simulink model "TSR_Scenario_003_cs"  (R2014b)
settings: Solver=ode5  SolverMode=SingleTasking  StartTime=0.0  StopTime=inf  FixedStep=1/100  RelTol=1e-3
PreLoadFcn:
  | mbxruntime.callbacks.PreLoadFcn(bdroot);
  | check_NUTS_defined;
  | 
  | assignin('base',['model_closed_' bdroot],false);
  | 
  | addpath('../includes_TSR/includes_TSR');
  | 
  | switch version('-release')
  | case {'2010a', '2010b', '2011a'}
  | addpath('../includes_TSR/ML2010b');
  | otherwise
  | addpath('../includes_TSR/ML2011b');
  | end
PostLoadFcn:
  | mbxruntime.callbacks.PostLoadFcn(bdroot);
InitFcn:
  | mbxruntime.callbacks.InitFcn(bdroot);
StartFcn:
  | mbxruntime.callbacks.StartFcn(bdroot);
StopFcn:
  | mbxruntime.callbacks.StopFcn(bdroot);
model workspace: external: MAT-File .\TSR_Scenario_003_cs_hws.mat (data not in the file)
undefined symbols (not defined in the file or in its folder): InitImageOutputDir, mbxruntime, OrientationPitch, OrientationRoll, PositionX, PositionY, PositionZ, tabledata, warningInitialVelocity, x0
undefined symbols (not defined in the file): SteeringColumn, SteeringWheel, TSR_Scenario_003_cs_031c08980fc50484, TSR_Scenario_003_cs_034f292ed02288d5, TSR_Scenario_003_cs_0459b3dfbc82c9a8, TSR_Scenario_003_cs_097620f815f21f1d, TSR_Scenario_003_cs_097d7573cc694bf5, TSR_Scenario_003_cs_0996a1a3dd5e2a3a, TSR_Scenario_003_cs_0f1849cdb4701326, TSR_Scenario_003_cs_10f4098912b3b5db, TSR_Scenario_003_cs_117f01ea831ec368, TSR_Scenario_003_cs_12cf78b79d36da1c, TSR_Scenario_003_cs_144fbb977118bf37, TSR_Scenario_003_cs_1523d5367c5052d0, TSR_Scenario_003_cs_1540f37e1ce5220e, TSR_Scenario_003_cs_15da4682074a9114, TSR_Scenario_003_cs_186e86d78e8adde8, TSR_Scenario_003_cs_198fefcb5c5d4c4a, TSR_Scenario_003_cs_1d24564a28ca8c57, TSR_Scenario_003_cs_1ea9b65b93b2d93e, TSR_Scenario_003_cs_1f4a4c0163bc654f, TSR_Scenario_003_cs_221c7f4f757b6f59, TSR_Scenario_003_cs_22229c9f69845439, TSR_Scenario_003_cs_230bf92302b3240a, TSR_Scenario_003_cs_23763ac742803108, TSR_Scenario_003_cs_237ee3c37f4d72b6, TSR_Scenario_003_cs_2956d712ba1268bc, TSR_Scenario_003_cs_2c8e6bdc42e74688, TSR_Scenario_003_cs_3037724928f99df0, TSR_Scenario_003_cs_31b44ca47ec5ff02, TSR_Scenario_003_cs_324745b613f45b9c, TSR_Scenario_003_cs_32b36e3fd4699b17, TSR_Scenario_003_cs_35d6077a5f3bdf8f, TSR_Scenario_003_cs_364710b5c901cafc, TSR_Scenario_003_cs_3727ee2f4430f2bb, TSR_Scenario_003_cs_382e41ab6806a13f, TSR_Scenario_003_cs_38ccddae174883be, TSR_Scenario_003_cs_3a0767dbf486e31b, TSR_Scenario_003_cs_3b460d19c10c747b, TSR_Scenario_003_cs_426c63b9f9c7abdf, TSR_Scenario_003_cs_42f1edf1b324bf4e, TSR_Scenario_003_cs_43b33e682c00a164, TSR_Scenario_003_cs_440a2f0d77aab01b, TSR_Scenario_003_cs_466378c5e179d625, TSR_Scenario_003_cs_4b8aa743d5bd8c1e, TSR_Scenario_003_cs_4bb095d5f4984042, TSR_Scenario_003_cs_4cec1a92176fe53d, TSR_Scenario_003_cs_4d6b6c843c52af2c, TSR_Scenario_003_cs_514fc139d324fd0d, TSR_Scenario_003_cs_51f4eff9e91179f9, TSR_Scenario_003_cs_56a9ea09cd860a89, TSR_Scenario_003_cs_5749c15298076949, TSR_Scenario_003_cs_576a8029b2a2792f, TSR_Scenario_003_cs_58b2f104991e8ca9, TSR_Scenario_003_cs_59a8a0af3bc025d5, TSR_Scenario_003_cs_5baf0e640050f43b, TSR_Scenario_003_cs_626299c795c4a86e, TSR_Scenario_003_cs_6499aa317499632d, TSR_Scenario_003_cs_676e881463a7df3e, TSR_Scenario_003_cs_68379cf1a8816ef6 ... (+115)
libraries: PreScanSimulinkLibrary x53, simulink_extras x37, simulink x29
(part 3 of 21)

== system TSR_Scenario_003_cs/Audi_A8_1_Indicator_front_right ==
  Audi_A8_1_Indicator_front_right : Inport  Tag=inport/IndicatorFR  OutDataTypeStr=Bus: PRESCAN_VISULIGHTACTUATOR_DATA  SampleTime=1/100  BusOutputAsStruct=on
  Actuator : S-Function  FunctionName=sfun_VisuLightActuator  Parameters=mbxruntime.parameters.convert(UniqueID), mbxruntime.parameters.convert(LightName), mbxruntime.parameters.convert(PivotName), mbxruntime.parameters.convert(TextureResources), mbxruntime.parameters.convert(ColorsObjectName), mbxruntime.parameters.convert(MeshOnColor), mbxruntime.parameters.convert(MeshOffColor),tabledata, TimeStep  EnableBusSupport=off  mask(PreScan Sink Block: VisuActiveLight){UniqueID=210, LightName=Audi_A8_1.LightActuator_8_IndicatorFR_ActiveLight, PivotName=Audi_A8_1.IndicatorFR_pivot, TextureResources={ '1' 'LightMap\HeadLight LB and HB.png' '2' 'LightMap\HeadLight LB.png' '3' 'LightMap\GeneralLight.png' '4' 'LightMap\BrakeLight.png'}, ColorsObjectName=Audi_A8_1.IndicatorFR, MeshOnColor=[255  165    0    0  255  165    0    0  102  102  102  255  510  420  178  255], MeshOffColor=[255  165    0    0  255  165    0    0  102  102  102  255    0    0    0  255], TimeStep=1/100}
      mask prompts: UniqueID "Parent Unique Identifier"; LightName "Light"; PivotName "Pivot"; TextureResources "Texture Resources"; ColorsObjectName "Light Fixture Color Object"; MeshOnColor "Light Fixture On Color"; MeshOffColor "Light Fixture Off Color"; TimeStep "Simulink time step"
      mask help:
      | The VisuActiveLight block provides a way for detailed animation of Light Sources, such as the indicator, brake, fog and main lights of a vehicle, or a light post.
      |
      | For more information, please click Help.
      mask init:
      | [tabledata] = mbxruntime.parameters.table(UniqueID,LightName,PivotName,TextureResources,ColorsObjectName,MeshOnColor,MeshOffColor);
      mask Help: eval('openHelp(209)')
      mask Display: image(imread('HeadLight.png'))
  wires:
  Audi_A8_1_Indicator_front_right/1 -> Actuator/1

== system TSR_Scenario_003_cs/Audi_A8_1_Indicator_rear_left ==
  Audi_A8_1_Indicator_rear_left : Inport  Tag=inport/IndicatorRL  OutDataTypeStr=Bus: PRESCAN_VISULIGHTACTUATOR_DATA  SampleTime=1/100  BusOutputAsStruct=on
  Actuator : S-Function  FunctionName=sfun_VisuLightActuator  Parameters=mbxruntime.parameters.convert(UniqueID), mbxruntime.parameters.convert(LightName), mbxruntime.parameters.convert(PivotName), mbxruntime.parameters.convert(TextureResources), mbxruntime.parameters.convert(ColorsObjectName), mbxruntime.parameters.convert(MeshOnColor), mbxruntime.parameters.convert(MeshOffColor),tabledata, TimeStep  EnableBusSupport=off  mask(PreScan Sink Block: VisuActiveLight){UniqueID=210, LightName=Audi_A8_1.LightActuator_7_IndicatorRL_ActiveLight, PivotName=Audi_A8_1.IndicatorRL_pivot, TextureResources={ '1' 'LightMap\HeadLight LB and HB.png' '2' 'LightMap\HeadLight LB.png' '3' 'LightMap\GeneralLight.png' '4' 'LightMap\BrakeLight.png'}, ColorsObjectName=Audi_A8_1.IndicatorRL, MeshOnColor=[255  165    0    0  255  165    0    0  102  102  102  255  510  420  178  255], MeshOffColor=[255  165    0    0  255  165    0    0  102  102  102  255    0    0    0  255], TimeStep=1/100}
      mask prompts: UniqueID "Parent Unique Identifier"; LightName "Light"; PivotName "Pivot"; TextureResources "Texture Resources"; ColorsObjectName "Light Fixture Color Object"; MeshOnColor "Light Fixture On Color"; MeshOffColor "Light Fixture Off Color"; TimeStep "Simulink time step"
      mask help:
      | The VisuActiveLight block provides a way for detailed animation of Light Sources, such as the indicator, brake, fog and main lights of a vehicle, or a light post.
      |
      | For more information, please click Help.
      mask init:
      | [tabledata] = mbxruntime.parameters.table(UniqueID,LightName,PivotName,TextureResources,ColorsObjectName,MeshOnColor,MeshOffColor);
      mask Help: eval('openHelp(209)')
      mask Display: image(imread('HeadLight.png'))
  wires:
  Audi_A8_1_Indicator_rear_left/1 -> Actuator/1

== system TSR_Scenario_003_cs/Audi_A8_1_Indicator_rear_right ==
  Audi_A8_1_Indicator_rear_right : Inport  Tag=inport/IndicatorRR  OutDataTypeStr=Bus: PRESCAN_VISULIGHTACTUATOR_DATA  SampleTime=1/100  BusOutputAsStruct=on
  Actuator : S-Function  FunctionName=sfun_VisuLightActuator  Parameters=mbxruntime.parameters.convert(UniqueID), mbxruntime.parameters.convert(LightName), mbxruntime.parameters.convert(PivotName), mbxruntime.parameters.convert(TextureResources), mbxruntime.parameters.convert(ColorsObjectName), mbxruntime.parameters.convert(MeshOnColor), mbxruntime.parameters.convert(MeshOffColor),tabledata, TimeStep  EnableBusSupport=off  mask(PreScan Sink Block: VisuActiveLight){UniqueID=210, LightName=Audi_A8_1.LightActuator_9_IndicatorRR_ActiveLight, PivotName=Audi_A8_1.IndicatorRR_pivot, TextureResources={ '1' 'LightMap\HeadLight LB and HB.png' '2' 'LightMap\HeadLight LB.png' '3' 'LightMap\GeneralLight.png' '4' 'LightMap\BrakeLight.png'}, ColorsObjectName=Audi_A8_1.IndicatorRR, MeshOnColor=[255  165    0    0  255  165    0    0  102  102  102  255  510  420  178  255], MeshOffColor=[255  165    0    0  255  165    0    0  102  102  102  255    0    0    0  255], TimeStep=1/100}
      mask prompts: UniqueID "Parent Unique Identifier"; LightName "Light"; PivotName "Pivot"; TextureResources "Texture Resources"; ColorsObjectName "Light Fixture Color Object"; MeshOnColor "Light Fixture On Color"; MeshOffColor "Light Fixture Off Color"; TimeStep "Simulink time step"
      mask help:
      | The VisuActiveLight block provides a way for detailed animation of Light Sources, such as the indicator, brake, fog and main lights of a vehicle, or a light post.
      |
      | For more information, please click Help.
      mask init:
      | [tabledata] = mbxruntime.parameters.table(UniqueID,LightName,PivotName,TextureResources,ColorsObjectName,MeshOnColor,MeshOffColor);
      mask Help: eval('openHelp(209)')
      mask Display: image(imread('HeadLight.png'))
  wires:
  Audi_A8_1_Indicator_rear_right/1 -> Actuator/1

== system TSR_Scenario_003_cs/BMW_X5_1 ==
  SELF_BMW_X5_1 : Inport  Tag=inport/SelfPort  OutDataTypeStr=Bus: PRESCAN_SELFSENSORDATA  PortDimensions=1  SampleTime=1/100  BusOutputAsStruct=on
  Dynamics_Empty : Subsystem  Tag=Dynamics_Empty
      mask Help: eval('openHelp(202)')
      mask Display: port_label('output', 1, 'State');text(0,0,' Empty\n')
  SELF_Demux : Subsystem  Tag=demux/SelfPort  mask(PreScan Demux Block:){}
      mask help:
      | The SELF port shows (state) information of the actor itself. The outputs are position in the experiment's axis system and the GPS coordinates, and the object's absolute velocity and compass heading.
      |
      | For more information, please click Help.
      settings: DeleteFcn=PreScanBlockDeleteFcn;
      mask Help: eval('openHelp(462)')
      mask Display:
      | port_label('output',1,'x [m]')
      | port_label('output',2,'y [m]')
      | port_label('output',3,'z [m]','texmode','on')
      | port_label('output',4,'Rotx [deg]','texmode','on')
      | port_label('output',5,'Roty [deg]','texmode','on')
      | port_label('output',6,'Rotz [deg]','texmode','on')
      | port_label('output',7,'GPS lat [deg]','texmode','on')
      | port_label('output',8,'GPS long [deg]','texmode','on')
      | port_label('output',9,'GPS alt [m]','texmode','on')
      | port_label('output',10,'Velocity [m/s]')
      | port_label('output',11,'Heading [deg]')
      | port_label('output',12,'Yaw rate [deg/s]')
  STATE_BMW_X5_1_rc : RateTransition  Tag=mux_rc/StatePort  OutPortSampleTimeOpt=Inherit
  Terminator_{1..12} (12 alike) : Terminator
  STATE_BMW_X5_1_bus : Outport  Tag=outport/StatePort  OutDataTypeStr=Bus: PRESCAN_STATEACTUATORDATA  PortDimensions=1  SampleTime=1/100
  wires:
  STATE_BMW_X5_1_rc/1 -> STATE_BMW_X5_1_bus/1
  Dynamics_Empty/1(State) -> STATE_BMW_X5_1_rc/1
  SELF_BMW_X5_1/1 -> SELF_Demux/1(SELF)
  SELF_Demux/1(x [m]) -> Terminator_1/1
  SELF_Demux/2(y [m]) -> Terminator_2/1
  SELF_Demux/3(z [m]) -> Terminator_3/1
  SELF_Demux/4(rotx [deg]) -> Terminator_4/1
  SELF_Demux/5(roty [deg]) -> Terminator_5/1
  SELF_Demux/6(rotz [deg]) -> Terminator_6/1
  SELF_Demux/7(GPS lat [deg]) -> Terminator_7/1
  SELF_Demux/8(GPS long [deg]) -> Terminator_8/1
  SELF_Demux/9(GPS alt [m]) -> Terminator_9/1
  SELF_Demux/10(velocity [m/s]) -> Terminator_10/1
  SELF_Demux/11(heading [deg]) -> Terminator_11/1
  SELF_Demux/12(yaw rate [deg/s]) -> Terminator_12/1

== system TSR_Scenario_003_cs/BMW_X5_2 ==
  SELF_BMW_X5_2 : Inport  Tag=inport/SelfPort  OutDataTypeStr=Bus: PRESCAN_SELFSENSORDATA  PortDimensions=1  SampleTime=1/100  BusOutputAsStruct=on
  Dynamics_Empty : Subsystem  Tag=Dynamics_Empty
      mask Help: eval('openHelp(202)')
      mask Display: port_label('output', 1, 'State');text(0,0,' Empty\n')
  SELF_Demux : Subsystem  Tag=demux/SelfPort  mask(PreScan Demux Block:){}
      mask help:
      | The SELF port shows (state) information of the actor itself. The outputs are position in the experiment's axis system and the GPS coordinates, and the object's absolute velocity and compass heading.
      |
      | For more information, please click Help.
      settings: DeleteFcn=PreScanBlockDeleteFcn;
      mask Help: eval('openHelp(462)')
      mask Display:
      | port_label('output',1,'x [m]')
      | port_label('output',2,'y [m]')
      | port_label('output',3,'z [m]','texmode','on')
      | port_label('output',4,'Rotx [deg]','texmode','on')
      | port_label('output',5,'Roty [deg]','texmode','on')
      | port_label('output',6,'Rotz [deg]','texmode','on')
      | port_label('output',7,'GPS lat [deg]','texmode','on')
      | port_label('output',8,'GPS long [deg]','texmode','on')
      | port_label('output',9,'GPS alt [m]','texmode','on')
      | port_label('output',10,'Velocity [m/s]')
      | port_label('output',11,'Heading [deg]')
      | port_label('output',12,'Yaw rate [deg/s]')
  STATE_BMW_X5_2_rc : RateTransition  Tag=mux_rc/StatePort  OutPortSampleTimeOpt=Inherit
  Terminator_{1..12} (12 alike) : Terminator
  STATE_BMW_X5_2_bus : Outport  Tag=outport/StatePort  OutDataTypeStr=Bus: PRESCAN_STATEACTUATORDATA  PortDimensions=1  SampleTime=1/100
  wires:
  STATE_BMW_X5_2_rc/1 -> STATE_BMW_X5_2_bus/1
  Dynamics_Empty/1(State) -> STATE_BMW_X5_2_rc/1
  SELF_BMW_X5_2/1 -> SELF_Demux/1(SELF)
  SELF_Demux/1(x [m]) -> Terminator_1/1
  SELF_Demux/2(y [m]) -> Terminator_2/1
  SELF_Demux/3(z [m]) -> Terminator_3/1
  SELF_Demux/4(rotx [deg]) -> Terminator_4/1
  SELF_Demux/5(roty [deg]) -> Terminator_5/1
  SELF_Demux/6(rotz [deg]) -> Terminator_6/1
  SELF_Demux/7(GPS lat [deg]) -> Terminator_7/1
  SELF_Demux/8(GPS long [deg]) -> Terminator_8/1
  SELF_Demux/9(GPS alt [m]) -> Terminator_9/1
  SELF_Demux/10(velocity [m/s]) -> Terminator_10/1
  SELF_Demux/11(heading [deg]) -> Terminator_11/1
  SELF_Demux/12(yaw rate [deg/s]) -> Terminator_12/1

== system TSR_Scenario_003_cs/BMW_X5_3 ==
  SELF_BMW_X5_3 : Inport  Tag=inport/SelfPort  OutDataTypeStr=Bus: PRESCAN_SELFSENSORDATA  PortDimensions=1  SampleTime=1/100  BusOutputAsStruct=on
  Dynamics_Empty : Subsystem  Tag=Dynamics_Empty
      mask Help: eval('openHelp(202)')
      mask Display: port_label('output', 1, 'State');text(0,0,' Empty\n')
  SELF_Demux : Subsystem  Tag=demux/SelfPort  mask(PreScan Demux Block:){}
      mask help:
      | The SELF port shows (state) information of the actor itself. The outputs are position in the experiment's axis system and the GPS coordinates, and the object's absolute velocity and compass heading.
      |
      | For more information, please click Help.
      settings: DeleteFcn=PreScanBlockDeleteFcn;
      mask Help: eval('openHelp(462)')
      mask Display:
      | port_label('output',1,'x [m]')
      | port_label('output',2,'y [m]')
      | port_label('output',3,'z [m]','texmode','on')
      | port_label('output',4,'Rotx [deg]','texmode','on')
      | port_label('output',5,'Roty [deg]','texmode','on')
      | port_label('output',6,'Rotz [deg]','texmode','on')
      | port_label('output',7,'GPS lat [deg]','texmode','on')
      | port_label('output',8,'GPS long [deg]','texmode','on')
      | port_label('output',9,'GPS alt [m]','texmode','on')
      | port_label('output',10,'Velocity [m/s]')
      | port_label('output',11,'Heading [deg]')
      | port_label('output',12,'Yaw rate [deg/s]')
  STATE_BMW_X5_3_rc : RateTransition  Tag=mux_rc/StatePort  OutPortSampleTimeOpt=Inherit
  Terminator_{1..12} (12 alike) : Terminator
  STATE_BMW_X5_3_bus : Outport  Tag=outport/StatePort  OutDataTypeStr=Bus: PRESCAN_STATEACTUATORDATA  PortDimensions=1  SampleTime=1/100
  wires:
  STATE_BMW_X5_3_rc/1 -> STATE_BMW_X5_3_bus/1
  Dynamics_Empty/1(State) -> STATE_BMW_X5_3_rc/1
  SELF_BMW_X5_3/1 -> SELF_Demux/1(SELF)
  SELF_Demux/1(x [m]) -> Terminator_1/1
  SELF_Demux/2(y [m]) -> Terminator_2/1
  SELF_Demux/3(z [m]) -> Terminator_3/1
  SELF_Demux/4(rotx [deg]) -> Terminator_4/1
  SELF_Demux/5(roty [deg]) -> Terminator_5/1
  SELF_Demux/6(rotz [deg]) -> Terminator_6/1
  SELF_Demux/7(GPS lat [deg]) -> Terminator_7/1
  SELF_Demux/8(GPS long [deg]) -> Terminator_8/1
  SELF_Demux/9(GPS alt [m]) -> Terminator_9/1
  SELF_Demux/10(velocity [m/s]) -> Terminator_10/1
  SELF_Demux/11(heading [deg]) -> Terminator_11/1
  SELF_Demux/12(yaw rate [deg/s]) -> Terminator_12/1

== system TSR_Scenario_003_cs/BMW_Z3_1 ==
  SELF_BMW_Z3_1 : Inport  Tag=inport/SelfPort  OutDataTypeStr=Bus: PRESCAN_SELFSENSORDATA  PortDimensions=1  SampleTime=1/100  BusOutputAsStruct=on
  Dynamics_Empty : Subsystem  Tag=Dynamics_Empty
      mask Help: eval('openHelp(202)')
      mask Display: port_label('output', 1, 'State');text(0,0,' Empty\n')
  SELF_Demux : Subsystem  Tag=demux/SelfPort  mask(PreScan Demux Block:){}
      mask help:
      | The SELF port shows (state) information of the actor itself. The outputs are position in the experiment's axis system and the GPS coordinates, and the object's absolute velocity and compass heading.
      |
      | For more information, please click Help.
      settings: DeleteFcn=PreScanBlockDeleteFcn;
      mask Help: eval('openHelp(462)')
      mask Display:
      | port_label('output',1,'x [m]')
      | port_label('output',2,'y [m]')
      | port_label('output',3,'z [m]','texmode','on')
      | port_label('output',4,'Rotx [deg]','texmode','on')
      | port_label('output',5,'Roty [deg]','texmode','on')
      | port_label('output',6,'Rotz [deg]','texmode','on')
      | port_label('output',7,'GPS lat [deg]','texmode','on')
      | port_label('output',8,'GPS long [deg]','texmode','on')
      | port_label('output',9,'GPS alt [m]','texmode','on')
      | port_label('output',10,'Velocity [m/s]')
      | port_label('output',11,'Heading [deg]')
      | port_label('output',12,'Yaw rate [deg/s]')
  STATE_BMW_Z3_1_rc : RateTransition  Tag=mux_rc/StatePort  OutPortSampleTimeOpt=Inherit
  Terminator_{1..12} (12 alike) : Terminator
  STATE_BMW_Z3_1_bus : Outport  Tag=outport/StatePort  OutDataTypeStr=Bus: PRESCAN_STATEACTUATORDATA  PortDimensions=1  SampleTime=1/100
  wires:
  STATE_BMW_Z3_1_rc/1 -> STATE_BMW_Z3_1_bus/1
  Dynamics_Empty/1(State) -> STATE_BMW_Z3_1_rc/1
  SELF_BMW_Z3_1/1 -> SELF_Demux/1(SELF)
  SELF_Demux/1(x [m]) -> Terminator_1/1
  SELF_Demux/2(y [m]) -> Terminator_2/1
  SELF_Demux/3(z [m]) -> Terminator_3/1
  SELF_Demux/4(rotx [deg]) -> Terminator_4/1
  SELF_Demux/5(roty [deg]) -> Terminator_5/1
  SELF_Demux/6(rotz [deg]) -> Terminator_6/1
  SELF_Demux/7(GPS lat [deg]) -> Terminator_7/1
  SELF_Demux/8(GPS long [deg]) -> Terminator_8/1
  SELF_Demux/9(GPS alt [m]) -> Terminator_9/1
  SELF_Demux/10(velocity [m/s]) -> Terminator_10/1
  SELF_Demux/11(heading [deg]) -> Terminator_11/1
  SELF_Demux/12(yaw rate [deg/s]) -> Terminator_12/1

== system TSR_Scenario_003_cs/CameraSensor_1 ==
  Sensor : S-Function  FunctionName=sfun_Camera  Parameters=sensorID, dataWidth, dataHeight, channelsPerImage, numberOfImages, timestep  EnableBusSupport=off  mask(PreScan Source Block: Camera Sensor){sensorID=239, dataWidth=600, dataHeight=2400, channelsPerImage=3, numberOfImages=1, timestep=1/50}
      mask prompts: sensorID "Sensor ID"; dataWidth "Data width"; dataHeight "Data Height"; channelsPerImage "Channels per image"; numberOfImages "Number of images"; timestep "MATLAB timestep:"
      mask help: The Camera Sensor provides a color or monochrome image.
      mask Help: eval('openHelp(457)')
      mask Display: image(imread('CameraSensor.png'))
  CameraSensor_1 : Outport  Tag=outport/Camera/CameraSensor  OutDataTypeStr=uint8  SampleTime=1/50
  wires:
  Sensor/1 -> CameraSensor_1/1

== system TSR_Scenario_003_cs/Citroen_C3_1 ==
  SELF_Citroen_C3_1 : Inport  Tag=inport/SelfPort  OutDataTypeStr=Bus: PRESCAN_SELFSENSORDATA  PortDimensions=1  SampleTime=1/100  BusOutputAsStruct=on
  Dynamics_Empty : Subsystem  Tag=Dynamics_Empty
      mask Help: eval('openHelp(202)')
      mask Display: port_label('output', 1, 'State');text(0,0,' Empty\n')
  SELF_Demux : Subsystem  Tag=demux/SelfPort  mask(PreScan Demux Block:){}
      mask help:
      | The SELF port shows (state) information of the actor itself. The outputs are position in the experiment's axis system and the GPS coordinates, and the object's absolute velocity and compass heading.
      |
      | For more information, please click Help.
      settings: DeleteFcn=PreScanBlockDeleteFcn;
      mask Help: eval('openHelp(462)')
      mask Display:
      | port_label('output',1,'x [m]')
      | port_label('output',2,'y [m]')
      | port_label('output',3,'z [m]','texmode','on')
      | port_label('output',4,'Rotx [deg]','texmode','on')
      | port_label('output',5,'Roty [deg]','texmode','on')
      | port_label('output',6,'Rotz [deg]','texmode','on')
      | port_label('output',7,'GPS lat [deg]','texmode','on')
      | port_label('output',8,'GPS long [deg]','texmode','on')
      | port_label('output',9,'GPS alt [m]','texmode','on')
      | port_label('output',10,'Velocity [m/s]')
      | port_label('output',11,'Heading [deg]')
      | port_label('output',12,'Yaw rate [deg/s]')
  STATE_Citroen_C3_1_rc : RateTransition  Tag=mux_rc/StatePort  OutPortSampleTimeOpt=Inherit
  Terminator_{1..12} (12 alike) : Terminator
  STATE_Citroen_C3_1_bus : Outport  Tag=outport/StatePort  OutDataTypeStr=Bus: PRESCAN_STATEACTUATORDATA  PortDimensions=1  SampleTime=1/100
  wires:
  STATE_Citroen_C3_1_rc/1 -> STATE_Citroen_C3_1_bus/1
  Dynamics_Empty/1(State) -> STATE_Citroen_C3_1_rc/1
  SELF_Citroen_C3_1/1 -> SELF_Demux/1(SELF)
  SELF_Demux/1(x [m]) -> Terminator_1/1
  SELF_Demux/2(y [m]) -> Terminator_2/1
  SELF_Demux/3(z [m]) -> Terminator_3/1
  SELF_Demux/4(rotx [deg]) -> Terminator_4/1
  SELF_Demux/5(roty [deg]) -> Terminator_5/1
  SELF_Demux/6(rotz [deg]) -> Terminator_6/1
  SELF_Demux/7(GPS lat [deg]) -> Terminator_7/1
  SELF_Demux/8(GPS long [deg]) -> Terminator_8/1
  SELF_Demux/9(GPS alt [m]) -> Terminator_9/1
  SELF_Demux/10(velocity [m/s]) -> Terminator_10/1
  SELF_Demux/11(heading [deg]) -> Terminator_11/1
  SELF_Demux/12(yaw rate [deg/s]) -> Terminator_12/1

== system TSR_Scenario_003_cs/Controller ==
  Terminator : Terminator
  sfun_Controller : S-Function  FunctionName=sfun_Controller  Parameters=SParameter1, SParameter2, SParameter3, SParameter4, SParameter5, SParameter6, SParameter7, SParameter8, SParameter9, SParameter10, SampleTime  EnableBusSupport=off  mask(Legacy Function){SFunctionSpec=void prescan_outputFcn(void** work1, PRESCAN_CONTROLLERDATA y1[1]), SParameter1=uint8([ExperimentFile 0]), SParameter2=uint8([ModelDepo 0]), SParameter3=uint8([ControllerOptions 0]), SParameter4=RTmode, SParameter5=PreScanExecutionMode, SParameter6=ControlMode, SParameter7=ControllerCount, SParameter8=ControllerIndex, SParameter9=uint8([SimulationMode 0]), SParameter10=uint8([TargetName 0]), SampleTime=TimeStep, ShowSpec=on}
      mask prompts: SParameter1 "P1:"; SParameter2 "P2:"; SParameter3 "P3:"; SParameter4 "P4:"; SParameter5 "P5:"; SParameter6 "P6:"; SParameter7 "P7:"; SParameter8 "P8:"; SParameter9 "P9:"; SParameter10 "P10:"; SampleTime "Sample time (-1 for inherited):"; ShowSpec "Display function specification"
      mask help:
      | This block allows you to call the legacy functions specified by the following Legacy Code Tool definition:
      | def.SFunctionName = 'sfun_Controller';
      | def.OutputFcnSpec = 'void prescan_outputFcn(void** work1, PRESCAN_CONTROLLERDATA y1[1])';
      | def.StartFcnSpec = 'void prescan_startFcn(void ** work1, uint8 p1[], uint8 p2[], uint8 p3[], double p4, double p5, double p6, double p7, double p8, uint8 p9[], uint8 p10[])';
      | def.TerminateFcnSpec = 'void prescan_terminateFcn(void** work1)';
      | def.HeaderFiles = {'prescan_controller_data.h', 'prescan_SFunLibrary.h', 'prescan_CreateLogHandler.h', 'prescan_CreateErrorHandler.h', 'prescan_modify.h', 'ModuleDLL.h'};
      | def.SourceFiles = {'prescan_MexLogHandler.c', 'prescan_SimStructErrorHandler.c', 'prescan_LogHandler.c', 'prescan_ErrorHandler.c', 'prescan_Modify.c'};
      | def.HostLibFiles = {'sensorinterfaced.lib'};
      | def.TargetLibFiles = {'sensorinterfaced.so'};
      | def.IncPaths = {'.', 'C:\projects\prescan\rt_vislibrary\vis\..\pimp\include\sensors\InterfaceRTW'};
      | def.SrcPaths = {'C:\projects\prescan\rt_vislibrary\vis\..\pimp\include\sensors\InterfaceRTW', 'C:\projects\prescan\rt_vislibrary\vis\..\pimp\include\sensors\InterfaceRTW\ccurrt'};
      | def.LibPaths = {'C:\\projects\\prescan\\vislibrary_build\lib'};
      | def.SampleTime = 'parameterized';
      mask Help: <p>This block was generated automatically by the Legacy Code Tool. For detailed help on this tool, call<a href="matlab:legacy_code('help')"> legacy_code('help')</a>.</p>
      mask Callback ShowSpec:
      | if strcmp(get_param(gcbh, 'ShowSpec'), 'on')
      |   set_param(gcbh, 'MaskDisplay', sprintf('fprintf(''%s'');', get_param(gcbh, 'SFunctionSpec')));
      | else
      |   set_param(gcbh, 'MaskDisplay', sprintf('fprintf(''%s'');', get_param(gcbh, 'FunctionName')));
      | end
      mask Display: fprintf('void prescan_outputFcn(void** work1, PRESCAN_CONTROLLERDATA y1[1])');
  wires:
  sfun_Controller/1 -> Terminator/1

== system TSR_Scenario_003_cs/Daf_95_1 ==
  SELF_Daf_95_1 : Inport  Tag=inport/SelfPort  OutDataTypeStr=Bus: PRESCAN_SELFSENSORDATA  PortDimensions=1  SampleTime=1/100  BusOutputAsStruct=on
  Path : S-Function  Tag=Path  LoadFcn=load('PrescanMotionData.mat')  FunctionName=sfun_Path  Parameters=uniqueID, pathUniqueID, timestep  EnableBusSupport=off  mask(Path){uniqueID=576, pathUniqueID=TSR_Scenario_003_cs_Daf_95_1_Path_pathUniqueID, timestep=1/100}
      mask prompts: uniqueID "Object Unique ID"; pathUniqueID "Path Unique ID"; timestep "MATLAB timestep:"
      mask help:
      | The path block outputs the position along a given trajectory.
      |
      | For more information, please click Help.
      mask Help: eval('openHelp(312)')
      mask Display: image(imread('Path.png'))
  SELF_Demux : Subsystem  Tag=demux/SelfPort  mask(PreScan Demux Block:){}
      mask help:
      | The SELF port shows (state) information of the actor itself. The outputs are position in the experiment's axis system and the GPS coordinates, and the object's absolute velocity and compass heading.
      |
      | For more information, please click Help.
      settings: DeleteFcn=PreScanBlockDeleteFcn;
      mask Help: eval('openHelp(462)')
      mask Display:
      | port_label('output',1,'x [m]')
      | port_label('output',2,'y [m]')
      | port_label('output',3,'z [m]','texmode','on')
      | port_label('output',4,'Rotx [deg]','texmode','on')
      | port_label('output',5,'Roty [deg]','texmode','on')
      | port_label('output',6,'Rotz [deg]','texmode','on')
      | port_label('output',7,'GPS lat [deg]','texmode','on')
      | port_label('output',8,'GPS long [deg]','texmode','on')
      | port_label('output',9,'GPS alt [m]','texmode','on')
      | port_label('output',10,'Velocity [m/s]')
      | port_label('output',11,'Heading [deg]')
      | port_label('output',12,'Yaw rate [deg/s]')
  STATE_Daf_95_1_rc : RateTransition  Tag=mux_rc/StatePort  OutPortSampleTimeOpt=Inherit
  SpeedProfile : S-Function  Tag=SpeedProfile  LoadFcn=load('PrescanMotionData.mat')  FunctionName=sfun_SpeedProfile  Parameters=speedProfileUniqueID, timestep  EnableBusSupport=off  mask(SpeedProfile){speedProfileUniqueID=TSR_Scenario_003_cs_Daf_95_1_SpeedProfile_speedProfileUniqueID, timestep=1/100}
      mask prompts: speedProfileUniqueID "Speed Profile Unique ID"; timestep "MATLAB timestep:"
      mask help:
      | The speed profile block outputs the travelled distance, velocities and acceleration along a given path.
      |
      | For more information, please click Help.
      mask Help: eval('openHelp(312)')
      mask Display: image(imread('SpeedProfile.png'))
  Terminator_{1..12} (12 alike) : Terminator
  STATE_Daf_95_1_bus : Outport  Tag=outport/StatePort  OutDataTypeStr=Bus: PRESCAN_STATEACTUATORDATA  PortDimensions=1  SampleTime=1/100
  wires:
  SpeedProfile/1 -> Path/1
  STATE_Daf_95_1_rc/1 -> STATE_Daf_95_1_bus/1
  Path/1 -> STATE_Daf_95_1_rc/1
  SELF_Daf_95_1/1 -> SELF_Demux/1(SELF)
  SELF_Demux/1(x [m]) -> Terminator_1/1
  SELF_Demux/2(y [m]) -> Terminator_2/1
  SELF_Demux/3(z [m]) -> Terminator_3/1
  SELF_Demux/4(rotx [deg]) -> Terminator_4/1
  SELF_Demux/5(roty [deg]) -> Terminator_5/1
  SELF_Demux/6(rotz [deg]) -> Terminator_6/1
  SELF_Demux/7(GPS lat [deg]) -> Terminator_7/1
  SELF_Demux/8(GPS long [deg]) -> Terminator_8/1
  SELF_Demux/9(GPS alt [m]) -> Terminator_9/1
  SELF_Demux/10(velocity [m/s]) -> Terminator_10/1
  SELF_Demux/11(heading [deg]) -> Terminator_11/1
  SELF_Demux/12(yaw rate [deg/s]) -> Terminator_12/1

== system TSR_Scenario_003_cs/Female_RegularAni_1 ==
  SELF_Female_RegularAni_1 : Inport  Tag=inport/SelfPort  OutDataTypeStr=Bus: PRESCAN_SELFSENSORDATA  PortDimensions=1  SampleTime=1/100  BusOutputAsStruct=on
  Animation : Subsystem  Tag=RunningHumanAnimation  mask(Prescan Conversion Block: Running Human Animation){MWS=1.95, WalkingScale=1.0, RunningScale=0.22, TimeStep=1/100}
      mask prompts: MWS "Maximum Walking Speed [m/s], above which the animation will switch to running mode."; WalkingScale "Walking mode scaling factor to sync the animation frames to the displacement."; RunningScale "Running mode scaling factor to sync the animation frames to the displacement."; TimeStep "Auto-Assigned: Upload Period [s]"
      mask help: The Running Human Animation block converts the State signal of a human into signals to properly control the animation.
      mask Help: eval('openHelp(239)');
      mask Display: image(imread('HumanAnimated.jpg'))
  ColorRegion_Lower_Body_color : Constant  Tag=VisuLightConst  Value=[0 0 0]
  ColorRegion_Shoes_color : Constant  Tag=VisuLightConst  Value=[255 255 255]
  ColorRegion_Upper_Body_color : Constant  Tag=VisuLightConst  Value=[0 255 255]
  Dynamics_Empty : Subsystem  Tag=Dynamics_Empty
      mask Help: eval('openHelp(202)')
      mask Display: port_label('output', 1, 'State');text(0,0,' Empty\n')
  SELF_Demux : Subsystem  Tag=demux/SelfPort  mask(PreScan Demux Block:){}
      mask help:
      | The SELF port shows (state) information of the actor itself. The outputs are position in the experiment's axis system and the GPS coordinates, and the object's absolute velocity and compass heading.
      |
      | For more information, please click Help.
      settings: DeleteFcn=PreScanBlockDeleteFcn;
      mask Help: eval('openHelp(462)')
      mask Display:
      | port_label('output',1,'x [m]')
      | port_label('output',2,'y [m]')
      | port_label('output',3,'z [m]','texmode','on')
      | port_label('output',4,'Rotx [deg]','texmode','on')
      | port_label('output',5,'Roty [deg]','texmode','on')
      | port_label('output',6,'Rotz [deg]','texmode','on')
      | port_label('output',7,'GPS lat [deg]','texmode','on')
      | port_label('output',8,'GPS long [deg]','texmode','on')
      | port_label('output',9,'GPS alt [m]','texmode','on')
      | port_label('output',10,'Velocity [m/s]')
      | port_label('output',11,'Heading [deg]')
      | port_label('output',12,'Yaw rate [deg/s]')
  STATE_Female_RegularAni_1_rc : RateTransition  Tag=mux_rc/StatePort  OutPortSampleTimeOpt=Inherit
  Terminator_{1..12} (12 alike) : Terminator
  VISUColorRegion_Lower_Body_Mux : Subsystem  Tag=mux/MuxColorRegion  LoadFcn=load PrescanColorData  mask(PreScan User Interface: VisuTextureColor){}
      mask help:
      | The VisuTextureColor block provides a way to adapt the color of a vehicle.
      |
      | For more information, please click Help.
      settings: DeleteFcn=PreScanBlockDeleteFcn;
      mask Help: eval('openHelp(230)')
  VISUColorRegion_Shoes_Mux : Subsystem  Tag=mux/MuxColorRegion  LoadFcn=load PrescanColorData  mask(PreScan User Interface: VisuTextureColor){}
      mask help:
      | The VisuTextureColor block provides a way to adapt the color of a vehicle.
      |
      | For more information, please click Help.
      settings: DeleteFcn=PreScanBlockDeleteFcn;
      mask Help: eval('openHelp(230)')
  VISUColorRegion_Upper_Body_Mux : Subsystem  Tag=mux/MuxColorRegion  LoadFcn=load PrescanColorData  mask(PreScan User Interface: VisuTextureColor){}
      mask help:
      | The VisuTextureColor block provides a way to adapt the color of a vehicle.
      |
      | For more information, please click Help.
      settings: DeleteFcn=PreScanBlockDeleteFcn;
      mask Help: eval('openHelp(230)')
  STATE_Female_RegularAni_1_bus : Outport  Tag=outport/StatePort  OutDataTypeStr=Bus: PRESCAN_STATEACTUATORDATA  PortDimensions=1  SampleTime=1/100
  ANIM_Female_RegularAni_1 : Outport  Tag=outport/AnimationOutport  Port=2  OutDataTypeStr=Bus: PRESCAN_ANIMACTUATORDATA  PortDimensions=1  SampleTime=1/100
  VISUColorRegion_Upper_Body_Female_RegularAni_1 : Outport  Tag=outport/ColorRegion  Port=3  OutDataTypeStr=Bus: PRESCAN_COLOR_DATA  PortDimensions=1  SampleTime=1/100
  VISUColorRegion_Lower_Body_Female_RegularAni_1 : Outport  Tag=outport/ColorRegion  Port=4  OutDataTypeStr=Bus: PRESCAN_COLOR_DATA  PortDimensions=1  SampleTime=1/100
  VISUColorRegion_Shoes_Female_RegularAni_1 : Outport  Tag=outport/ColorRegion  Port=5  OutDataTypeStr=Bus: PRESCAN_COLOR_DATA  PortDimensions=1  SampleTime=1/100
  wires:
  STATE_Female_RegularAni_1_rc/1 -> STATE_Female_RegularAni_1_bus/1
  Dynamics_Empty/1(State) -> STATE_Female_RegularAni_1_rc/1, Animation/1(In1)
  Animation/1(Out1) -> ANIM_Female_RegularAni_1/1
  SELF_Female_RegularAni_1/1 -> SELF_Demux/1(SELF)
  VISUColorRegion_Upper_Body_Mux/1(ColorRegion) -> VISUColorRegion_Upper_Body_Female_RegularAni_1/1
  ColorRegion_Upper_Body_color/1 -> VISUColorRegion_Upper_Body_Mux/1(RGB [-,-,-])
  VISUColorRegion_Lower_Body_Mux/1(ColorRegion) -> VISUColorRegion_Lower_Body_Female_RegularAni_1/1
  ColorRegion_Lower_Body_color/1 -> VISUColorRegion_Lower_Body_Mux/1(RGB [-,-,-])
  VISUColorRegion_Shoes_Mux/1(ColorRegion) -> VISUColorRegion_Shoes_Female_RegularAni_1/1
  ColorRegion_Shoes_color/1 -> VISUColorRegion_Shoes_Mux/1(RGB [-,-,-])
  SELF_Demux/1(x [m]) -> Terminator_1/1
  SELF_Demux/2(y [m]) -> Terminator_2/1
  SELF_Demux/3(z [m]) -> Terminator_3/1
  SELF_Demux/4(rotx [deg]) -> Terminator_4/1
  SELF_Demux/5(roty [deg]) -> Terminator_5/1
  SELF_Demux/6(rotz [deg]) -> Terminator_6/1
  SELF_Demux/7(GPS lat [deg]) -> Terminator_7/1
  SELF_Demux/8(GPS long [deg]) -> Terminator_8/1
  SELF_Demux/9(GPS alt [m]) -> Terminator_9/1
  SELF_Demux/10(velocity [m/s]) -> Terminator_10/1
  SELF_Demux/11(heading [deg]) -> Terminator_11/1
  SELF_Demux/12(yaw rate [deg/s]) -> Terminator_12/1

== system TSR_Scenario_003_cs/Female_Regular_wBuggy_1 ==
  SELF_Female_Regular_wBuggy_1 : Inport  Tag=inport/SelfPort  OutDataTypeStr=Bus: PRESCAN_SELFSENSORDATA  PortDimensions=1  SampleTime=1/100  BusOutputAsStruct=on
  Animation : Subsystem  Tag=WalkingHumanAnimation  mask(Prescan Conversion Block: Walking Human Animation){TimeStep=1/100}
      mask prompts: TimeStep "Auto-Assigned: Upload Period [s]"
      mask help: The Walking Human Animation block converts the State signal of a human into signals to properly control the animation.
      mask Help: eval('openHelp(239)');
      mask Display: image(imread('HumanAnimated.jpg'))
  ColorRegion_Lower_Body_color : Constant  Tag=VisuLightConst  Value=[220 20 60]
  ColorRegion_Shoes_color : Constant  Tag=VisuLightConst  Value=[0 0 0]
  ColorRegion_Upper_Body_color : Constant  Tag=VisuLightConst  Value=[185 209 234]
  Dynamics_Empty : Subsystem  Tag=Dynamics_Empty
      mask Help: eval('openHelp(202)')
      mask Display: port_label('output', 1, 'State');text(0,0,' Empty\n')
  SELF_Demux : Subsystem  Tag=demux/SelfPort  mask(PreScan Demux Block:){}
      mask help:
      | The SELF port shows (state) information of the actor itself. The outputs are position in the experiment's axis system and the GPS coordinates, and the object's absolute velocity and compass heading.
      |
      | For more information, please click Help.
      settings: DeleteFcn=PreScanBlockDeleteFcn;
      mask Help: eval('openHelp(462)')
      mask Display:
      | port_label('output',1,'x [m]')
      | port_label('output',2,'y [m]')
      | port_label('output',3,'z [m]','texmode','on')
      | port_label('output',4,'Rotx [deg]','texmode','on')
      | port_label('output',5,'Roty [deg]','texmode','on')
      | port_label('output',6,'Rotz [deg]','texmode','on')
      | port_label('output',7,'GPS lat [deg]','texmode','on')
      | port_label('output',8,'GPS long [deg]','texmode','on')
      | port_label('output',9,'GPS alt [m]','texmode','on')
      | port_label('output',10,'Velocity [m/s]')
      | port_label('output',11,'Heading [deg]')
      | port_label('output',12,'Yaw rate [deg/s]')
  STATE_Female_Regular_wBuggy_1_rc : RateTransition  Tag=mux_rc/StatePort  OutPortSampleTimeOpt=Inherit
  Terminator_{1..12} (12 alike) : Terminator
  VISUColorRegion_Lower_Body_Mux : Subsystem  Tag=mux/MuxColorRegion  LoadFcn=load PrescanColorData  mask(PreScan User Interface: VisuTextureColor){}
      mask help:
      | The VisuTextureColor block provides a way to adapt the color of a vehicle.
      |
      | For more information, please click Help.
      settings: DeleteFcn=PreScanBlockDeleteFcn;
      mask Help: eval('openHelp(230)')
  VISUColorRegion_Shoes_Mux : Subsystem  Tag=mux/MuxColorRegion  LoadFcn=load PrescanColorData  mask(PreScan User Interface: VisuTextureColor){}
      mask help:
      | The VisuTextureColor block provides a way to adapt the color of a vehicle.
      |
      | For more information, please click Help.
      settings: DeleteFcn=PreScanBlockDeleteFcn;
      mask Help: eval('openHelp(230)')
  VISUColorRegion_Upper_Body_Mux : Subsystem  Tag=mux/MuxColorRegion  LoadFcn=load PrescanColorData  mask(PreScan User Interface: VisuTextureColor){}
      mask help:
      | The VisuTextureColor block provides a way to adapt the color of a vehicle.
      |
      | For more information, please click Help.
      settings: DeleteFcn=PreScanBlockDeleteFcn;
      mask Help: eval('openHelp(230)')
  STATE_Female_Regular_wBuggy_1_bus : Outport  Tag=outport/StatePort  OutDataTypeStr=Bus: PRESCAN_STATEACTUATORDATA  PortDimensions=1  SampleTime=1/100
  ANIM_Female_Regular_wBuggy_1 : Outport  Tag=outport/AnimationOutport  Port=2  OutDataTypeStr=Bus: PRESCAN_ANIMACTUATORDATA  PortDimensions=1  SampleTime=1/100
  VISUColorRegion_Upper_Body_Female_Regular_wBuggy_1 : Outport  Tag=outport/ColorRegion  Port=3  OutDataTypeStr=Bus: PRESCAN_COLOR_DATA  PortDimensions=1  SampleTime=1/100
  VISUColorRegion_Lower_Body_Female_Regular_wBuggy_1 : Outport  Tag=outport/ColorRegion  Port=4  OutDataTypeStr=Bus: PRESCAN_COLOR_DATA  PortDimensions=1  SampleTime=1/100
  VISUColorRegion_Shoes_Female_Regular_wBuggy_1 : Outport  Tag=outport/ColorRegion  Port=5  OutDataTypeStr=Bus: PRESCAN_COLOR_DATA  PortDimensions=1  SampleTime=1/100
  wires:
  STATE_Female_Regular_wBuggy_1_rc/1 -> STATE_Female_Regular_wBuggy_1_bus/1
  Dynamics_Empty/1(State) -> STATE_Female_Regular_wBuggy_1_rc/1, Animation/1(In1)
  Animation/1(Out1) -> ANIM_Female_Regular_wBuggy_1/1
  SELF_Female_Regular_wBuggy_1/1 -> SELF_Demux/1(SELF)
  VISUColorRegion_Upper_Body_Mux/1(ColorRegion) -> VISUColorRegion_Upper_Body_Female_Regular_wBuggy_1/1
  ColorRegion_Upper_Body_color/1 -> VISUColorRegion_Upper_Body_Mux/1(RGB [-,-,-])
  VISUColorRegion_Lower_Body_Mux/1(ColorRegion) -> VISUColorRegion_Lower_Body_Female_Regular_wBuggy_1/1
  ColorRegion_Lower_Body_color/1 -> VISUColorRegion_Lower_Body_Mux/1(RGB [-,-,-])
  VISUColorRegion_Shoes_Mux/1(ColorRegion) -> VISUColorRegion_Shoes_Female_Regular_wBuggy_1/1
  ColorRegion_Shoes_color/1 -> VISUColorRegion_Shoes_Mux/1(RGB [-,-,-])
  SELF_Demux/1(x [m]) -> Terminator_1/1
  SELF_Demux/2(y [m]) -> Terminator_2/1
  SELF_Demux/3(z [m]) -> Terminator_3/1
  SELF_Demux/4(rotx [deg]) -> Terminator_4/1
  SELF_Demux/5(roty [deg]) -> Terminator_5/1
  SELF_Demux/6(rotz [deg]) -> Terminator_6/1
  SELF_Demux/7(GPS lat [deg]) -> Terminator_7/1
  SELF_Demux/8(GPS long [deg]) -> Terminator_8/1
  SELF_Demux/9(GPS alt [m]) -> Terminator_9/1
  SELF_Demux/10(velocity [m/s]) -> Terminator_10/1
  SELF_Demux/11(heading [deg]) -> Terminator_11/1
  SELF_Demux/12(yaw rate [deg/s]) -> Terminator_12/1

== system TSR_Scenario_003_cs/Fiat_Bravo_1 ==
  SELF_Fiat_Bravo_1 : Inport  Tag=inport/SelfPort  OutDataTypeStr=Bus: PRESCAN_SELFSENSORDATA  PortDimensions=1  SampleTime=1/100  BusOutputAsStruct=on
  Dynamics_Empty : Subsystem  Tag=Dynamics_Empty
      mask Help: eval('openHelp(202)')
      mask Display: port_label('output', 1, 'State');text(0,0,' Empty\n')
  SELF_Demux : Subsystem  Tag=demux/SelfPort  mask(PreScan Demux Block:){}
      mask help:
      | The SELF port shows (state) information of the actor itself. The outputs are position in the experiment's axis system and the GPS coordinates, and the object's absolute velocity and compass heading.
      |
      | For more information, please click Help.
      settings: DeleteFcn=PreScanBlockDeleteFcn;
      mask Help: eval('openHelp(462)')
      mask Display:
      | port_label('output',1,'x [m]')
      | port_label('output',2,'y [m]')
      | port_label('output',3,'z [m]','texmode','on')
      | port_label('output',4,'Rotx [deg]','texmode','on')
      | port_label('output',5,'Roty [deg]','texmode','on')
      | port_label('output',6,'Rotz [deg]','texmode','on')
      | port_label('output',7,'GPS lat [deg]','texmode','on')
      | port_label('output',8,'GPS long [deg]','texmode','on')
      | port_label('output',9,'GPS alt [m]','texmode','on')
      | port_label('output',10,'Velocity [m/s]')
      | port_label('output',11,'Heading [deg]')
      | port_label('output',12,'Yaw rate [deg/s]')
  STATE_Fiat_Bravo_1_rc : RateTransition  Tag=mux_rc/StatePort  OutPortSampleTimeOpt=Inherit
  Terminator_{1..12} (12 alike) : Terminator
  STATE_Fiat_Bravo_1_bus : Outport  Tag=outport/StatePort  OutDataTypeStr=Bus: PRESCAN_STATEACTUATORDATA  PortDimensions=1  SampleTime=1/100
  wires:
  STATE_Fiat_Bravo_1_rc/1 -> STATE_Fiat_Bravo_1_bus/1
  Dynamics_Empty/1(State) -> STATE_Fiat_Bravo_1_rc/1
  SELF_Fiat_Bravo_1/1 -> SELF_Demux/1(SELF)
  SELF_Demux/1(x [m]) -> Terminator_1/1
  SELF_Demux/2(y [m]) -> Terminator_2/1
  SELF_Demux/3(z [m]) -> Terminator_3/1
  SELF_Demux/4(rotx [deg]) -> Terminator_4/1
  SELF_Demux/5(roty [deg]) -> Terminator_5/1
  SELF_Demux/6(rotz [deg]) -> Terminator_6/1
  SELF_Demux/7(GPS lat [deg]) -> Terminator_7/1
  SELF_Demux/8(GPS long [deg]) -> Terminator_8/1
  SELF_Demux/9(GPS alt [m]) -> Terminator_9/1
  SELF_Demux/10(velocity [m/s]) -> Terminator_10/1
  SELF_Demux/11(heading [deg]) -> Terminator_11/1
  SELF_Demux/12(yaw rate [deg/s]) -> Terminator_12/1

== system TSR_Scenario_003_cs/Fiat_Bravo_2 ==
  SELF_Fiat_Bravo_2 : Inport  Tag=inport/SelfPort  OutDataTypeStr=Bus: PRESCAN_SELFSENSORDATA  PortDimensions=1  SampleTime=1/100  BusOutputAsStruct=on
  Dynamics_Empty : Subsystem  Tag=Dynamics_Empty
      mask Help: eval('openHelp(202)')
      mask Display: port_label('output', 1, 'State');text(0,0,' Empty\n')
  SELF_Demux : Subsystem  Tag=demux/SelfPort  mask(PreScan Demux Block:){}
      mask help:
      | The SELF port shows (state) information of the actor itself. The outputs are position in the experiment's axis system and the GPS coordinates, and the object's absolute velocity and compass heading.
      |
      | For more information, please click Help.
      settings: DeleteFcn=PreScanBlockDeleteFcn;
      mask Help: eval('openHelp(462)')
      mask Display:
      | port_label('output',1,'x [m]')
      | port_label('output',2,'y [m]')
      | port_label('output',3,'z [m]','texmode','on')
      | port_label('output',4,'Rotx [deg]','texmode','on')
      | port_label('output',5,'Roty [deg]','texmode','on')
      | port_label('output',6,'Rotz [deg]','texmode','on')
      | port_label('output',7,'GPS lat [deg]','texmode','on')
      | port_label('output',8,'GPS long [deg]','texmode','on')
      | port_label('output',9,'GPS alt [m]','texmode','on')
      | port_label('output',10,'Velocity [m/s]')
      | port_label('output',11,'Heading [deg]')
      | port_label('output',12,'Yaw rate [deg/s]')
  STATE_Fiat_Bravo_2_rc : RateTransition  Tag=mux_rc/StatePort  OutPortSampleTimeOpt=Inherit
  Terminator_{1..12} (12 alike) : Terminator
  STATE_Fiat_Bravo_2_bus : Outport  Tag=outport/StatePort  OutDataTypeStr=Bus: PRESCAN_STATEACTUATORDATA  PortDimensions=1  SampleTime=1/100
  wires:
  STATE_Fiat_Bravo_2_rc/1 -> STATE_Fiat_Bravo_2_bus/1
  Dynamics_Empty/1(State) -> STATE_Fiat_Bravo_2_rc/1
  SELF_Fiat_Bravo_2/1 -> SELF_Demux/1(SELF)
  SELF_Demux/1(x [m]) -> Terminator_1/1
  SELF_Demux/2(y [m]) -> Terminator_2/1
  SELF_Demux/3(z [m]) -> Terminator_3/1
  SELF_Demux/4(rotx [deg]) -> Terminator_4/1
  SELF_Demux/5(roty [deg]) -> Terminator_5/1
  SELF_Demux/6(rotz [deg]) -> Terminator_6/1
  SELF_Demux/7(GPS lat [deg]) -> Terminator_7/1
  SELF_Demux/8(GPS long [deg]) -> Terminator_8/1
  SELF_Demux/9(GPS alt [m]) -> Terminator_9/1
  SELF_Demux/10(velocity [m/s]) -> Terminator_10/1
  SELF_Demux/11(heading [deg]) -> Terminator_11/1
  SELF_Demux/12(yaw rate [deg/s]) -> Terminator_12/1
